simulink library "dlbsBlockBceLoss"  (R2025b)
settings: Solver=VariableStepAuto  StartTime=0.0  StopTime=10.0  RelTol=1e-3
libraries: dlbsBlockAdd x3, dlbsBlockGain x3, dlbsBlockExtractGradientGF x2, dlbsBlockLog x2, dlbsBlockProduct x2, dlbsBlockSplit x2, dlbsBlockInsertGradientGF x1, dlbsBlockMean x1
settings Model: Creator=lt6037  LastModifiedBy=lt6037

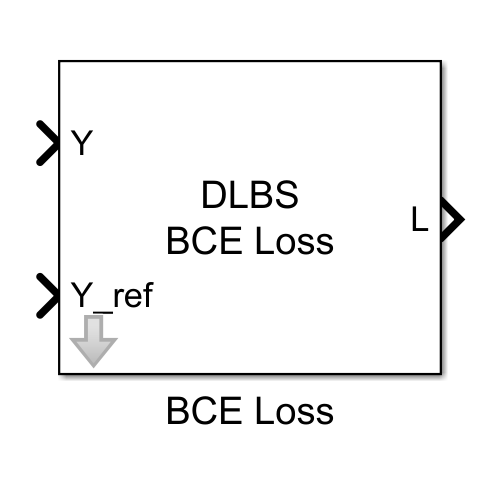
[thumbnail: Simulink's stored preview of the top-level diagram]
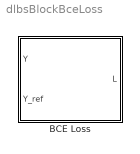
== system dlbsBlockBceLoss ==
  BCE Loss : Subsystem
      mask help: The Binary Cross-Entropy (BCE) Loss block computes the element-wise binary cross-entropy between a prediction tensor and a reference tensor, and outputs a scalar loss value.
      mask Help: web("dlbsHelpBlockBceLoss.html")
      mask Display: fprintf("DLBS\nBCE Loss")

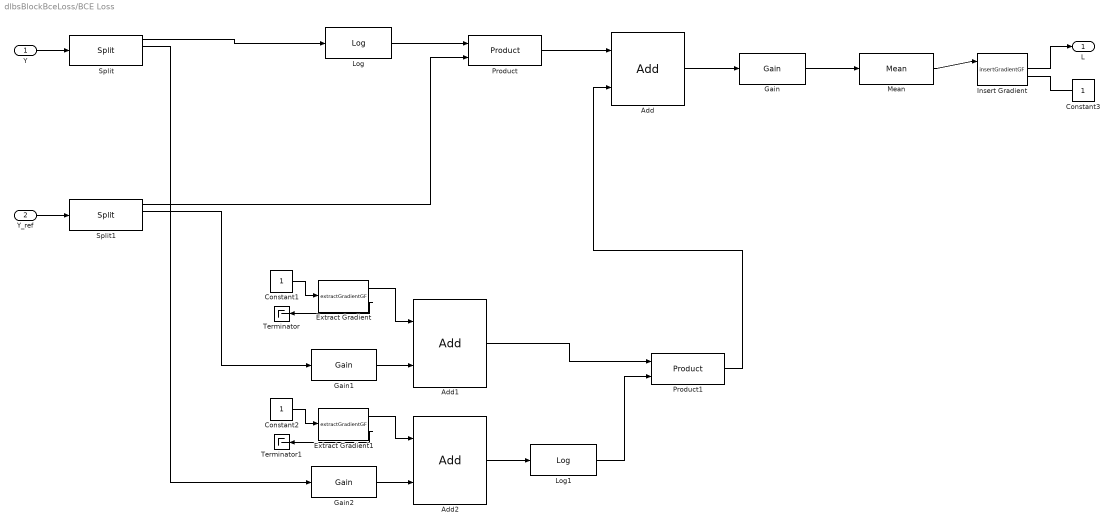
== system dlbsBlockBceLoss/BCE Loss ==
  Y : Inport
  Y_ref : Inport  Port=2
  Add : dlbsBlockAdd/Add  LabelModeActiveChoice=no broadcast  broadcast=off  dims1=1  dims2=1
  Add1 : dlbsBlockAdd/Add  LabelModeActiveChoice=no broadcast  broadcast=off  dims1=1  dims2=1
  Add2 : dlbsBlockAdd/Add  LabelModeActiveChoice=no broadcast  broadcast=off  dims1=1  dims2=1
  Constant1 : Constant
  Constant2 : Constant
  Constant3 : Constant
  Extract Gradient : dlbsBlockExtractGradientGF/extractGradientGF
  Extract Gradient1 : dlbsBlockExtractGradientGF/extractGradientGF
  Gain : dlbsBlockGain/Gain  Gain=-1
  Gain1 : dlbsBlockGain/Gain  Gain=-1
  Gain2 : dlbsBlockGain/Gain  Gain=-1
  Insert Gradient : dlbsBlockInsertGradientGF/insertGradientGF
  Log : dlbsBlockLog/Log
  Log1 : dlbsBlockLog/Log
  Mean : dlbsBlockMean/Mean
  Product : dlbsBlockProduct/Product
  Product1 : dlbsBlockProduct/Product
  Split : dlbsBlockSplit/Split  n_out=2  g1=on  g2=on  g3=on  g4=on
  Split1 : dlbsBlockSplit/Split  n_out=2  g1=on  g2=on  g3=on  g4=on
  Terminator : Terminator
  Terminator1 : Terminator
  L : Outport
  wires:
  Insert Gradient/1 -> L/1
  Constant3/1 -> Insert Gradient/2
  Constant1/1 -> Extract Gradient/1
  Extract Gradient/2 -> Terminator/1
  Constant2/1 -> Extract Gradient1/1
  Extract Gradient1/2 -> Terminator1/1
  Split/1 -> Log/1
  Split/2 -> Gain2/1
  Log/1 -> Product/1
  Product/1 -> Add/1
  Add/1 -> Gain/1
  Gain/1 -> Mean/1
  Mean/1 -> Insert Gradient/1
  Split1/1 -> Product/2
  Split1/2 -> Gain1/1
  Gain1/1 -> Add1/2
  Extract Gradient/1 -> Add1/1
  Gain2/1 -> Add2/2
  Extract Gradient1/1 -> Add2/1
  Add1/1 -> Product1/1
  Add2/1 -> Log1/1
  Log1/1 -> Product1/2
  Product1/1 -> Add/2
  Y/1 -> Split/1
  Y_ref/1 -> Split1/1
